simulink model "experiment"  (R2017a)
settings: Solver=ode3  StartTime=0.0  StopTime=inf  FixedStep=Ts_sim  RelTol=1e-3  EnableMultiTasking=on
model workspace (MAT data in the model file):
  SL_ROS_VariableLengthArrays_MaxSizes.CommonInfo.ArrayTruncateAction = 'EmitWarning'
  SL_ROS_VariableLengthArrays_MaxSizes.MsgTypeMap = containers.Map
  SL_ROS_VariableLengthArrays_MaxSizes.MsgTypeMap.serialization.keys = {'std_msgs/Int16MultiArray'}
  SL_ROS_VariableLengthArrays_MaxSizes.MsgTypeMap.serialization.values{1}.PropertyName = 'Data'
  SL_ROS_VariableLengthArrays_MaxSizes.MsgTypeMap.serialization.values{1}.DataType = 'int16'
  SL_ROS_VariableLengthArrays_MaxSizes.MsgTypeMap.serialization.values{1}.MaxLength = 2
  SL_ROS_VariableLengthArrays_MaxSizes.MsgTypeMap.serialization.uniformity = 0
  SL_ROS_VariableLengthArrays_MaxSizes.MsgTypeMap.serialization.keyType = 'char'
  SL_ROS_VariableLengthArrays_MaxSizes.MsgTypeMap.serialization.valueType = 'any'
values from neighbouring files (symbols this model uses):
  b_stop = 2*J*omega_n_stop*xsi_stop    [initializeParameters.m]
  delta_EMG_RT = double(max(EMG_vect_calRT)-min(EMG_vect_calRT))    [initializeParameters.m]
  delta_theta1 = thetaR1_rest - pi/2    (= 0.0728705481978)    [initializeParameters.m]
  EMG2vel_gain = 1*pi    (= 3.14159265359)    [initializeParameters.m]
  emgConst2 = 0    [initializeParameters.m]
  g = 9.81    [initializeParameters.m]
  input_type = 2    [initializeParameters.m]
  k_stop = J*omega_n_stop^2    [initializeParameters.m]
  Ki_vel = 0.75    [initializeParameters.m]
  Kp_vel = 7.5    [initializeParameters.m]
  L_com = tau_lift/(-m_arm*g*cos(thetaR1_lift - delta_theta1))    [initializeParameters.m]
  m1 = (y2_1-y1_1)/(x2_1-x1_1)    (= -1)    [initializeParameters.m]
  m3 = (y2_3-y1_3)/(x2_3-x1_3)    (= -1)    [initializeParameters.m]
  m_arm = 3.45    [initializeParameters.m]
  min_EMG_RT = double(min(EMG_vect_calRT))    [initializeParameters.m]
  q1 = -x1_1*m1 + y1_1    (= 90)    [initializeParameters.m]
  q3 = -x1_3*m3 + y1_3    (= 90)    [initializeParameters.m]
  tau_max_cont = 21    [initializeParameters.m]
  thetaL1_max = 70/180*pi    (= 1.2217304764)    [initializeParameters.m]
  thetaL1_min = -70/180*pi    (= -1.2217304764)    [initializeParameters.m]
  thetaR1_max = 70/180*pi    (= 1.2217304764)    [initializeParameters.m]
  thetaR1_min = -70/180*pi    (= -1.2217304764)    [initializeParameters.m]
undefined symbols (not defined in the file or in its folder): A_butter_cal, A_butter_low, B_butter_cal, B_butter_low, robotics, X, Y, Z
libraries: sm_lib x16, nesl_utility x7, robotlib x3
settings Model: ExtModeTrigDuration=2  Creator=Fred Parietti  LastModifiedBy=jacob
settings DataIOCC: LimitDataPoints=on  SaveFormat=Array
settings OptimizationCC: LifeSpan=1
settings DebuggingCC: UnderspecifiedInitializationDetection=Classic  MergeDetectMultiDrivingBlocksExec=none  SFUnexpectedBacktrackingDiag=warning  SFNoUnconditionalDefaultTransitionDiag=warning  SFExecutionAtInitializationDiag=none
settings HardwareCC: ProdBitPerInt=16  ProdBitPerPointer=8  ProdBitPerSizeT=16  ProdBitPerPtrDiffT=16  ProdLargestAtomicFloat=None  ProdWordSize=8  ProdHWDeviceType=Atmel->AVR
settings ModelReferenceCC: PropagateSignalLabelsOutOfModel=off
settings SFSimCC: MATLABDynamicMemAlloc=off
settings RTWCC: SystemTargetFile=realtime.tlc  GenerateMakefile=off  TemplateMakefile=realtime.tmf  Description=Run on Target Hardware  RTWVerbose=off
settings STFCustomTargetCC: TargetLibSuffix=.a  GenerateSampleERTMain=on  ERTCustomFileBanners=on  SupportNonInlinedSFcns=off  RemoveResetFunc=on  SupportVariableSizeSignals=on  MATLABClassNameForMDSCustomization=Simulink.SoftwareTarget.ERTCustomization  GRTInterface=off  SystemTargetFile=realtime.tlc
settings ERTTargetCC: MultiwordLength=2048  GenerateSampleERTMain=on  ParMdlRefBuildCompliant=off  CompOptLevelCompliant=off  ConcurrentExecutionCompliant=off  CombineOutputUpdateFcns=off  ERTFirstTimeCompliant=off  SupportContinuousTime=on  SupportVariableSizeSignals=on  ModelStepFunctionPrototypeControlCompliant=off  CPPClassGenCompliant=off  UseToolchainInfoCompliant=off  ExtModeTransport=3  ExtModeMexFile=ext_serial_win32_comm_rtt  ExtModeMexArgs=0 1 9600  ERTSrcFileBannerTemplate=realtime_code_template.cgt  ERTHdrFileBannerTemplate=realtime_code_template.cgt  ERTDataSrcFileTemplate=realtime_code_template.cgt  ERTDataHdrFileTemplate=realtime_code_template.cgt  ERTCustomFileTemplate=realtime_file_process.tlc  ConvertIfToSwitch=off  SuppressUnreachableDefaultCases=off
settings ConfigComp: CovMetricSettings=dw  CovHtmlReporting=on  CovSaveCumulativeToWorkspaceVar=on  CovSaveSingleToWorkspaceVar=on  CovExternalEMLEnable=off

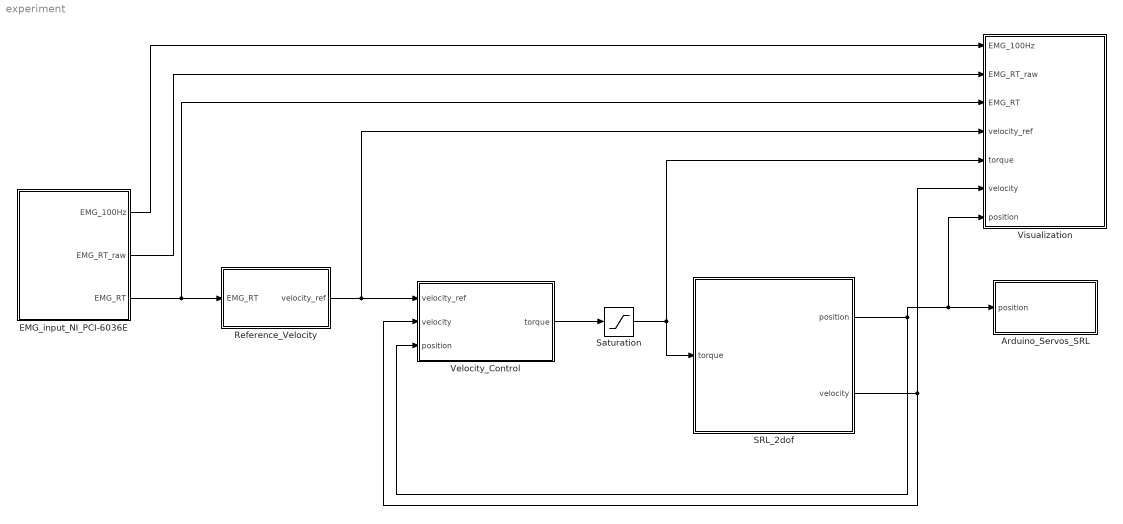
== system experiment ==
  Arduino_Servos_SRL : Subsystem  LoadFcn=robotics.ros.createSimulinkBus(gcs);
  EMG_input_NI_PCI-6036E : Subsystem
  Reference_Velocity : Subsystem
  SRL_2dof : Subsystem
  Saturation : Saturate  UpperLimit=tau_max_cont  LowerLimit=-tau_max_cont
  Velocity_Control : Subsystem
  Visualization : Subsystem
  wires:
  SRL_2dof/1(position) -> Visualization/7(position), Arduino_Servos_SRL/1(position), Velocity_Control/3(position)
  Saturation/1 -> Visualization/5(torque), SRL_2dof/1(torque)
  SRL_2dof/2(velocity) -> Visualization/6(velocity), Velocity_Control/2(velocity)
  Reference_Velocity/1(velocity_ref) -> Velocity_Control/1(velocity_ref), Visualization/4(velocity_ref)
  Velocity_Control/1(torque) -> Saturation/1
  EMG_input_NI_PCI-6036E/3(EMG_RT) -> Visualization/3(EMG_RT), Reference_Velocity/1(EMG_RT)
  EMG_input_NI_PCI-6036E/2(EMG_RT_raw) -> Visualization/2(EMG_RT_raw)
  EMG_input_NI_PCI-6036E/1(EMG_100Hz) -> Visualization/1(EMG_100Hz)

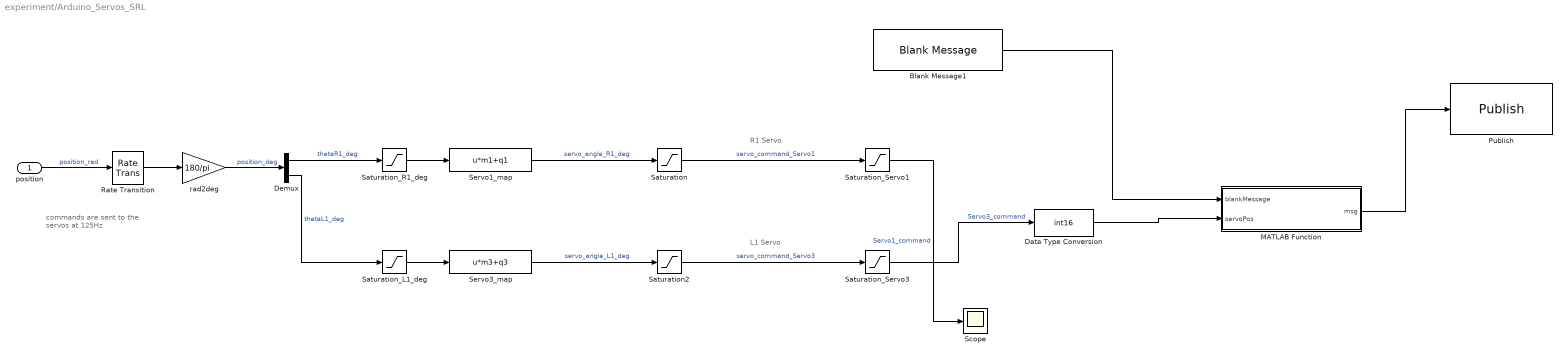
== system experiment/Arduino_Servos_SRL ==
  note: R1 Servo
  note: L1 Servo
  note: commands are sent to the servos at 125Hz
  position : Inport
  Blank Message1 : robotlib/Blank Message  SourceLibraryInfo=This block requires Robotics System Toolbox  messageType=std_msgs/Int16  SampleTime=inf
      settings: SourceProductBaseCode=RO
  Data Type Conversion : DataTypeConversion  OutDataTypeStr=int16  RndMeth=Round
  Demux : Demux  Outputs=2
  MATLAB Function : MATLAB Function  TreatAsAtomicUnit=on
  Publish : robotlib/Publish  SourceLibraryInfo=This block requires Robotics System Toolbox  topicSource=Specify your own  topic=/servoPosEMG  messageType=std_msgs/Int16  messageQueueLength=1
      settings: SourceProductBaseCode=RO
  Rate Transition : RateTransition  Deterministic=off  OutPortSampleTime=0.008
  Saturation : Saturate  UpperLimit=150  LowerLimit=23
  Saturation2 : Saturate  UpperLimit=158  LowerLimit=30
  Saturation_L1_deg : Saturate  UpperLimit=thetaL1_max/pi*180  LowerLimit=thetaL1_min/pi*180
  Saturation_R1_deg : Saturate  UpperLimit=thetaR1_max/pi*180  LowerLimit=thetaR1_min/pi*180
  Saturation_Servo1 : Saturate  UpperLimit=180  LowerLimit=0
  Saturation_Servo3 : Saturate  UpperLimit=180  LowerLimit=0
  Scope : Scope
  Servo1_map : Fcn  Expr=u*m1+q1
  Servo3_map : Fcn  Expr=u*m3+q3
  rad2deg : Gain  Gain=180/pi
  wires:
  position/1 -> Rate Transition/1  "position_rad"
  rad2deg/1 -> Demux/1  "position_deg"
  Demux/1 -> Saturation_R1_deg/1  "thetaR1_deg"
  Servo1_map/1 -> Saturation/1  "servo_angle_R1_deg"
  Demux/2 -> Saturation_L1_deg/1  "thetaL1_deg"
  Servo3_map/1 -> Saturation2/1  "servo_angle_L1_deg"
  Rate Transition/1 -> rad2deg/1
  Saturation/1 -> Saturation_Servo1/1  "servo_command_Servo1"
  Saturation2/1 -> Saturation_Servo3/1  "servo_command_Servo3"
  Saturation_R1_deg/1 -> Servo1_map/1
  Saturation_L1_deg/1 -> Servo3_map/1
  Blank Message1/1 -> MATLAB Function/1(blankMessage)
  Data Type Conversion/1 -> MATLAB Function/2(servoPos)
  MATLAB Function/1(msg) -> Publish/1
  Saturation_Servo3/1 -> Data Type Conversion/1  "Servo3_command"
  Saturation_Servo1/1 -> Scope/1  "Servo1_command"

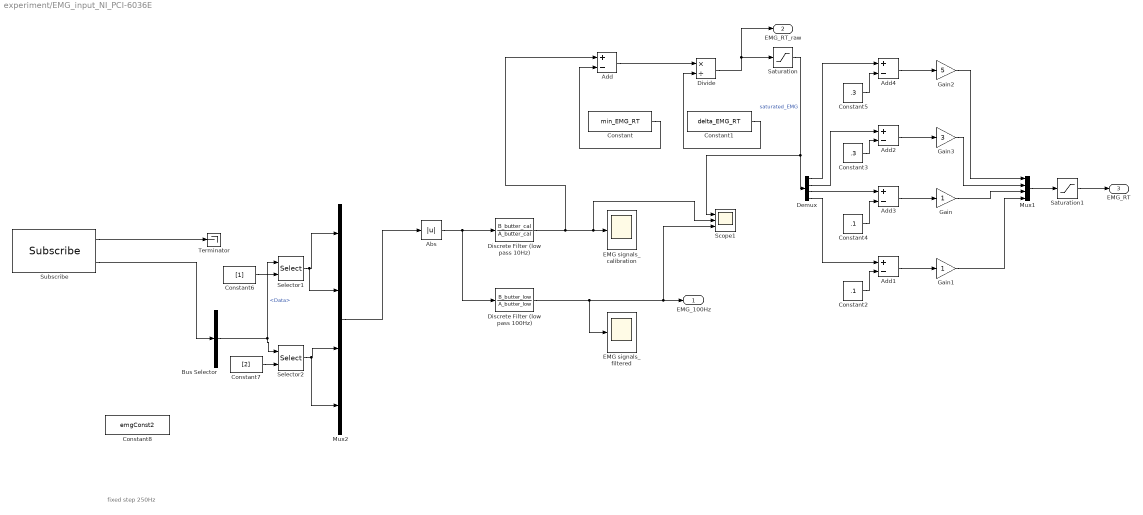
== system experiment/EMG_input_NI_PCI-6036E ==
  note: fixed step 250Hz
  Abs : Abs
  Add{,1..4} (5 alike) : Sum  Inputs=+-
  Bus Selector : BusSelector  OutputSignals=Data
  Constant : Constant  Value=min_EMG_RT
  Constant1 : Constant  Value=delta_EMG_RT
  Constant2 : Constant  Value=.1
  Constant3 : Constant  Value=.3
  Constant4 : Constant  Value=.1
  Constant5 : Constant  Value=.3
  Constant6 : Constant  Value=[1]
  Constant7 : Constant  Value=[2]
  Constant8 : Constant  Value=emgConst2  VectorParams1D=off  OutDataTypeStr=int16
  Demux : Demux
  Discrete Filter (low pass 100Hz) : DiscreteFilter  Numerator=B_butter_low  Denominator=A_butter_low
  Discrete Filter (low pass 10Hz) : DiscreteFilter  Numerator=B_butter_cal  Denominator=A_butter_cal
  Divide : Product  Inputs=*/
  EMG signals_calibration : Scope
  EMG signals_filtered : Scope
  Gain : Gain
  Gain1 : Gain
  Gain2 : Gain  Gain=5
  Gain3 : Gain  Gain=3
  Mux1 : Mux
  Mux2 : Mux
  Saturation : Saturate  UpperLimit=1  LowerLimit=0
  Saturation1 : Saturate  UpperLimit=1  LowerLimit=0
  Scope1 : Scope  NumInputPorts=3
  Selector1 : Selector  IndexOptions=Index vector (port)  Indices=[1 3]  OutputSizes=1
  Selector2 : Selector  IndexOptions=Index vector (port)  Indices=[1 3]  OutputSizes=1
  Subscribe : robotlib/Subscribe  SourceLibraryInfo=This block requires Robotics System Toolbox  topicSource=Select from ROS network  topic=/emgPub  messageType=std_msgs/Int16MultiArray  sampleTime=-1  messageQueueLength=1
      settings: SourceProductBaseCode=RO
  Terminator : Terminator
  EMG_100Hz : Outport
  EMG_RT_raw : Outport  Port=2
  EMG_RT : Outport  Port=3
  wires:
  Constant/1 -> Add/2
  Add/1 -> Divide/1
  Constant1/1 -> Divide/2
  Saturation/1 -> Scope1/1, Demux/1  "saturated_EMG"
  Demux/4 -> Add1/1
  Constant2/1 -> Add1/2
  Demux/1 -> Add4/1
  Add1/1 -> Gain1/1
  Mux1/1 -> Saturation1/1
  Demux/2 -> Add2/1
  Constant3/1 -> Add2/2
  Add2/1 -> Gain3/1
  Saturation1/1 -> EMG_RT/1
  Demux/3 -> Add3/1
  Add3/1 -> Gain/1
  Constant4/1 -> Add3/2
  Constant5/1 -> Add4/2
  Add4/1 -> Gain2/1
  Gain/1 -> Mux1/3
  Gain1/1 -> Mux1/4
  Gain2/1 -> Mux1/1
  Gain3/1 -> Mux1/2
  Discrete Filter (low pass 10Hz)/1 -> Add/1, Scope1/2, EMG signals_calibration/1
  Mux2/1 -> Abs/1
  Abs/1 -> Discrete Filter (low pass 10Hz)/1, Discrete Filter (low pass 100Hz)/1
  Divide/1 -> EMG_RT_raw/1, Saturation/1
  Discrete Filter (low pass 100Hz)/1 -> Scope1/3, EMG_100Hz/1, EMG signals_filtered/1
  Selector2/1 -> Mux2/4, Mux2/3
  Bus Selector/1 -> Selector2/1, Selector1/1  "<Data>"
  Subscribe/2 -> Bus Selector/1
  Constant6/1 -> Selector1/2
  Constant7/1 -> Selector2/2
  Subscribe/1 -> Terminator/1
  Selector1/1 -> Mux2/2, Mux2/1

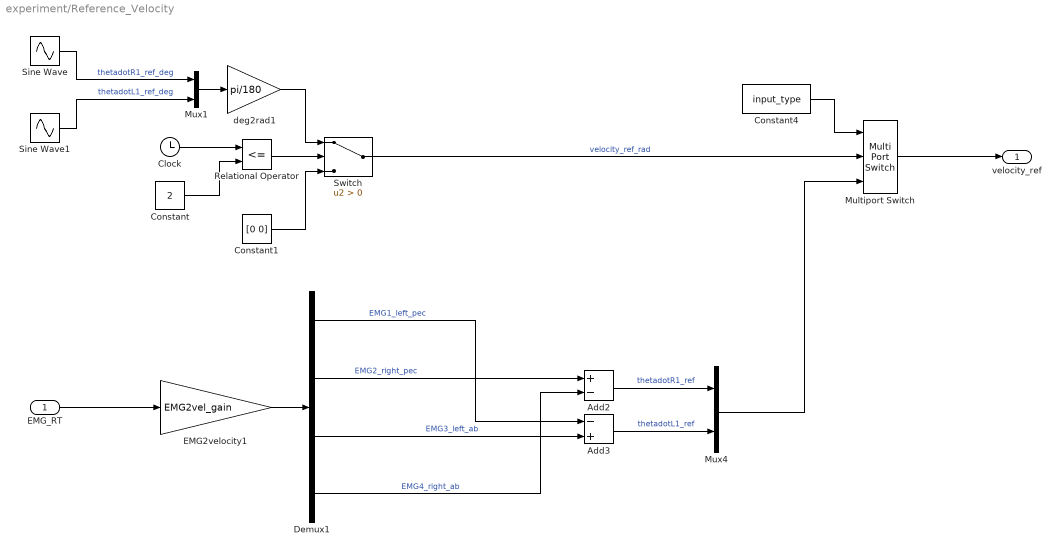
== system experiment/Reference_Velocity ==
  EMG_RT : Inport
  Add2 : Sum  Inputs=+-
  Add3 : Sum  Inputs=-+
  Clock : Clock
  Constant : Constant  Value=2
  Constant1 : Constant  Value=[0 0]
  Constant4 : Constant  Value=input_type
  Demux1 : Demux
  EMG2velocity1 : Gain  Gain=EMG2vel_gain
  Multiport Switch : MultiPortSwitch  Inputs=2
  Mux1 : Mux  Inputs=2
  Mux4 : Mux  Inputs=2
  Relational Operator : RelationalOperator  Operator=<=  OutDataTypeStr=boolean  RndMeth=Nearest
  Sine Wave : Sin  Amplitude=-40  Frequency=2*pi/(4)  SampleTime=0
  Sine Wave1 : Sin  Amplitude=-40  Frequency=2*pi/(4)  SampleTime=0
  Switch : Switch  Criteria=u2 > Threshold
  deg2rad1 : Gain  Gain=pi/180
  velocity_ref : Outport
  wires:
  Sine Wave/1 -> Mux1/1  "thetadotR1_ref_deg"
  Mux1/1 -> deg2rad1/1
  Switch/1 -> Multiport Switch/2  "velocity_ref_rad"
  Clock/1 -> Relational Operator/1
  Constant1/1 -> Switch/3
  Constant/1 -> Relational Operator/2
  Relational Operator/1 -> Switch/2
  deg2rad1/1 -> Switch/1
  Sine Wave1/1 -> Mux1/2  "thetadotL1_ref_deg"
  Constant4/1 -> Multiport Switch/1
  Multiport Switch/1 -> velocity_ref/1
  EMG2velocity1/1 -> Demux1/1
  Demux1/1 -> Add3/1  "EMG1_left_pec"
  Demux1/2 -> Add2/1  "EMG2_right_pec"
  Demux1/3 -> Add3/2  "EMG3_left_ab"
  Demux1/4 -> Add2/2  "EMG4_right_ab"
  Add2/1 -> Mux4/1  "thetadotR1_ref"
  Add3/1 -> Mux4/2  "thetadotL1_ref"
  EMG_RT/1 -> EMG2velocity1/1
  Mux4/1 -> Multiport Switch/3

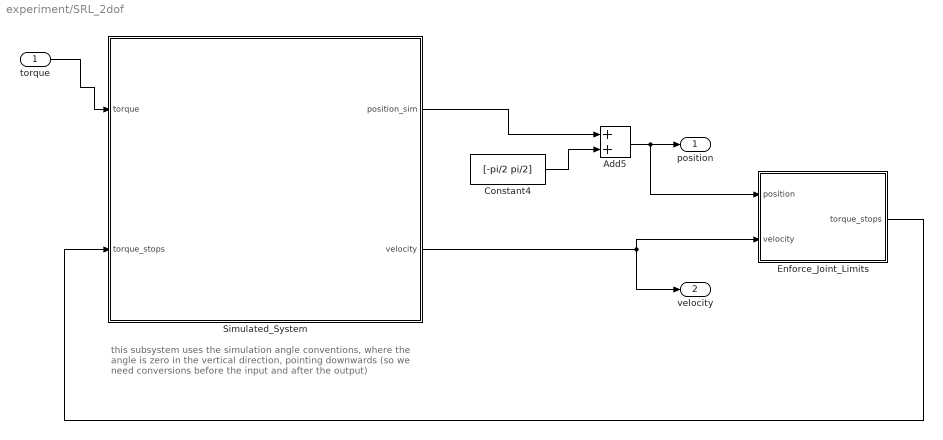
== system experiment/SRL_2dof ==
  note: this subsystem uses the simulation angle conventions, where the
      | angle is zero in the vertical direction, pointing downwards
      | (so we need conversions before the input and after the output)
  torque : Inport
  Add5 : Sum
  Constant4 : Constant  Value=[-pi/2 pi/2]
  Enforce_Joint_Limits : Subsystem
  Simulated_System : Subsystem
  position : Outport
  velocity : Outport  Port=2
  wires:
  Constant4/1 -> Add5/2
  Simulated_System/2(velocity) -> Enforce_Joint_Limits/2(velocity), velocity/1
  torque/1 -> Simulated_System/1(torque)
  Enforce_Joint_Limits/1(torque_stops) -> Simulated_System/2(torque_stops)
  Simulated_System/1(position_sim) -> Add5/1
  Add5/1 -> Enforce_Joint_Limits/1(position), position/1

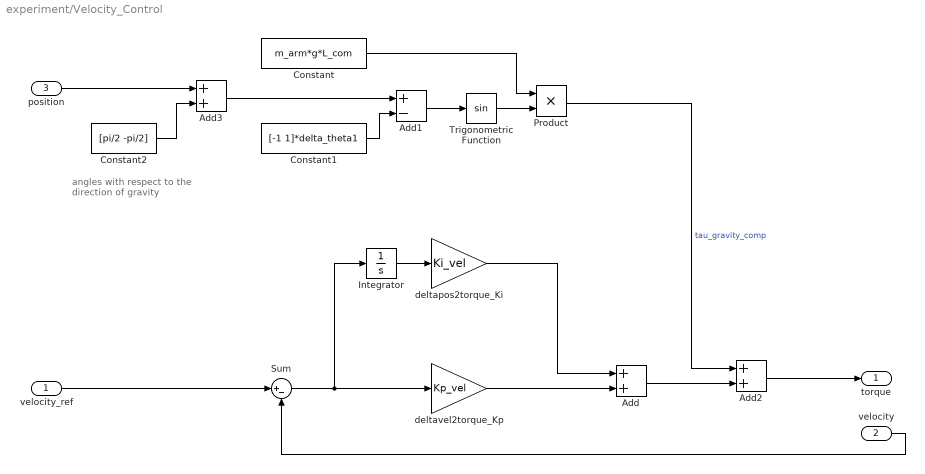
== system experiment/Velocity_Control ==
  note: angles with respect to
      | the direction of gravity
  velocity_ref : Inport
  velocity : Inport  Port=2
  position : Inport  Port=3
  Add : Sum
  Add1 : Sum  Inputs=+-
  Add2 : Sum
  Add3 : Sum
  Constant : Constant  Value=m_arm*g*L_com
  Constant1 : Constant  Value=[-1 1]*delta_theta1
  Constant2 : Constant  Value=[pi/2 -pi/2]
  Integrator : Integrator
  Product : Product
  Sum : Sum  Inputs=|+-
  Trigonometric Function : Trigonometry
  deltapos2torque_Ki : Gain  Gain=Ki_vel
  deltavel2torque_Kp : Gain  Gain=Kp_vel
  torque : Outport
  wires:
  velocity_ref/1 -> Sum/1
  velocity/1 -> Sum/2
  Sum/1 -> deltavel2torque_Kp/1, Integrator/1
  deltavel2torque_Kp/1 -> Add/2
  deltapos2torque_Ki/1 -> Add/1
  Add/1 -> Add2/2
  Integrator/1 -> deltapos2torque_Ki/1
  position/1 -> Add3/1
  Constant1/1 -> Add1/2
  Add1/1 -> Trigonometric Function/1
  Constant/1 -> Product/1
  Trigonometric Function/1 -> Product/2
  Product/1 -> Add2/1  "tau_gravity_comp"
  Add2/1 -> torque/1
  Add3/1 -> Add1/1
  Constant2/1 -> Add3/2

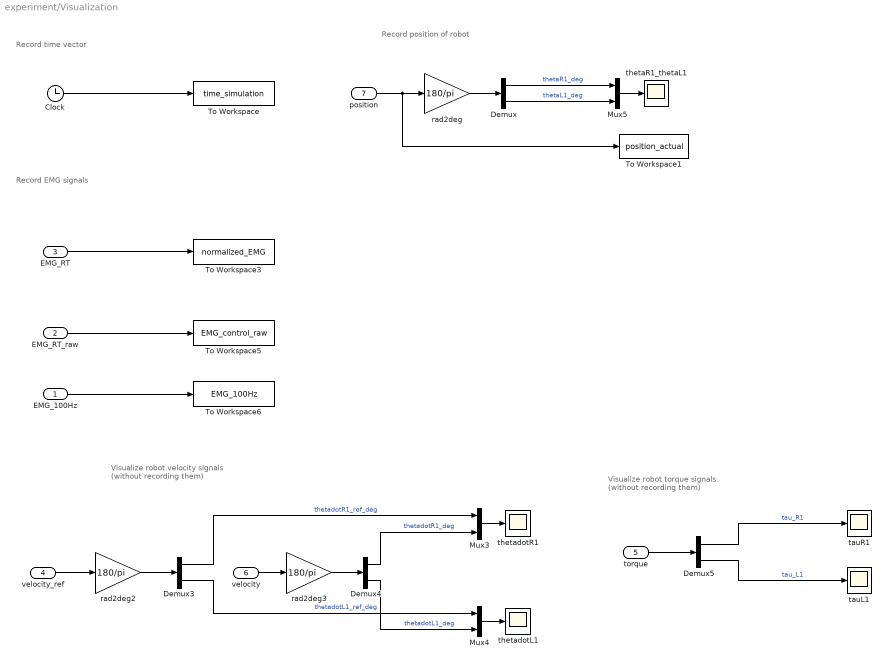
== system experiment/Visualization ==
  note: Record position of robot
  note: Record time vector
  note: Record EMG signals
  note: Visualize robot velocity signals (without recording them)
  note: Visualize robot torque signals (without recording them)
  EMG_100Hz : Inport
  EMG_RT_raw : Inport  Port=2
  EMG_RT : Inport  Port=3
  velocity_ref : Inport  Port=4
  torque : Inport  Port=5
  velocity : Inport  Port=6
  position : Inport  Port=7
  Clock : Clock
  Demux{,3..5} (4 alike) : Demux  Outputs=2
  Mux3 : Mux  Inputs=2
  Mux4 : Mux  Inputs=2
  Mux5 : Mux  Inputs=2
  To Workspace : ToWorkspace  VariableName=time_simulation  SampleTime=-1
  To Workspace1 : ToWorkspace  VariableName=position_actual  SampleTime=-1
  To Workspace3 : ToWorkspace  VariableName=normalized_EMG  SampleTime=-1
  To Workspace5 : ToWorkspace  VariableName=EMG_control_raw  SampleTime=-1
  To Workspace6 : ToWorkspace  VariableName=EMG_100Hz  SampleTime=-1
  rad2deg : Gain  Gain=180/pi
  rad2deg2 : Gain  Gain=180/pi
  rad2deg3 : Gain  Gain=180/pi
  tauL1 : Scope
  tauR1 : Scope
  thetaR1_thetaL1 : Scope
  thetadotL1 : Scope
  thetadotR1 : Scope
  wires:
  torque/1 -> Demux5/1
  Demux5/2 -> tauL1/1  "tau_L1"
  Demux5/1 -> tauR1/1  "tau_R1"
  velocity_ref/1 -> rad2deg2/1
  rad2deg2/1 -> Demux3/1
  velocity/1 -> rad2deg3/1
  Mux3/1 -> thetadotR1/1
  Demux3/1 -> Mux3/1  "thetadotR1_ref_deg"
  rad2deg3/1 -> Demux4/1
  Demux4/1 -> Mux3/2  "thetadotR1_deg"
  Mux4/1 -> thetadotL1/1
  Demux4/2 -> Mux4/2  "thetadotL1_deg"
  Demux3/2 -> Mux4/1  "thetadotL1_ref_deg"
  Clock/1 -> To Workspace/1
  EMG_RT/1 -> To Workspace3/1
  EMG_RT_raw/1 -> To Workspace5/1
  EMG_100Hz/1 -> To Workspace6/1
  position/1 -> rad2deg/1, To Workspace1/1
  rad2deg/1 -> Demux/1
  Demux/2 -> Mux5/2  "thetaL1_deg"
  Demux/1 -> Mux5/1  "thetaR1_deg"
  Mux5/1 -> thetaR1_thetaL1/1

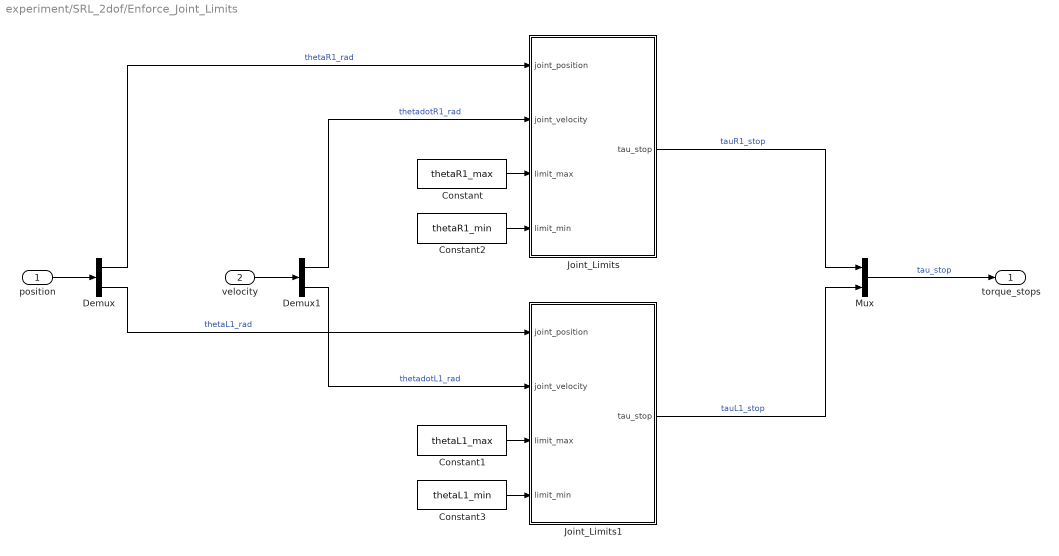
== system experiment/SRL_2dof/Enforce_Joint_Limits ==
  position : Inport
  velocity : Inport  Port=2
  Constant : Constant  Value=thetaR1_max
  Constant1 : Constant  Value=thetaL1_max
  Constant2 : Constant  Value=thetaR1_min
  Constant3 : Constant  Value=thetaL1_min
  Demux : Demux  Outputs=2
  Demux1 : Demux  Outputs=2
  Joint_Limits : Subsystem
  Joint_Limits1 : Subsystem
  Mux : Mux  Inputs=2
  torque_stops : Outport
  wires:
  position/1 -> Demux/1
  velocity/1 -> Demux1/1
  Demux1/1 -> Joint_Limits/2(joint_velocity)  "thetadotR1_rad"
  Constant/1 -> Joint_Limits/3(limit_max)
  Demux/1 -> Joint_Limits/1(joint_position)  "thetaR1_rad"
  Constant2/1 -> Joint_Limits/4(limit_min)
  Joint_Limits/1(tau_stop) -> Mux/1  "tauR1_stop"
  Mux/1 -> torque_stops/1  "tau_stop"
  Demux1/2 -> Joint_Limits1/2(joint_velocity)  "thetadotL1_rad"
  Demux/2 -> Joint_Limits1/1(joint_position)  "thetaL1_rad"
  Constant1/1 -> Joint_Limits1/3(limit_max)
  Constant3/1 -> Joint_Limits1/4(limit_min)
  Joint_Limits1/1(tau_stop) -> Mux/2  "tauL1_stop"

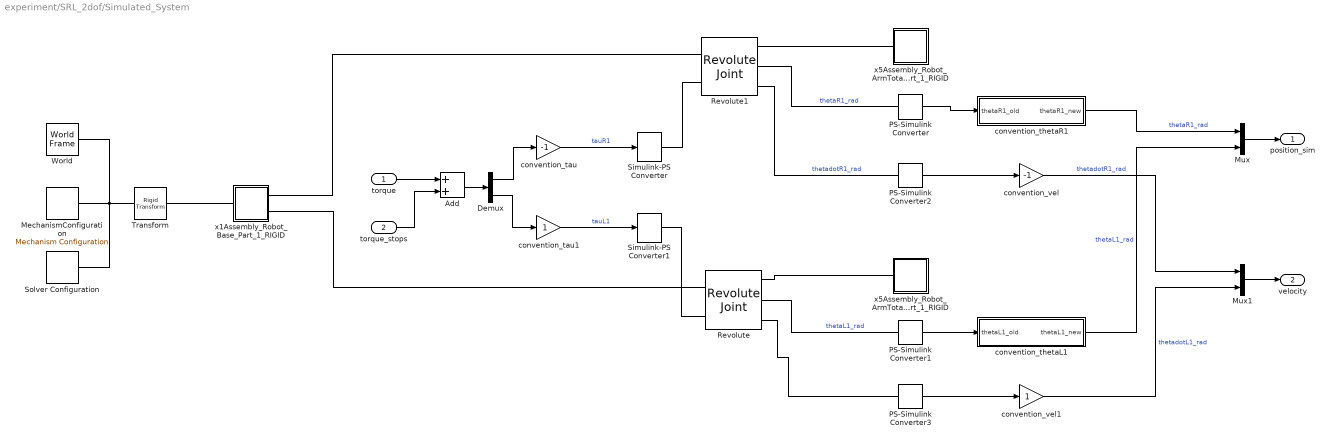
== system experiment/SRL_2dof/Simulated_System ==
  torque : Inport
  torque_stops : Inport  Port=2
  Add : Sum
  Demux : Demux  Outputs=2
  MechanismConfiguration : sm_lib/Utilities/Mechanism Configuration  UniformGravity=Constant  GravityVector=[0 -9.81 0]  GravityUnits=m/s^2  LinearizationDelta=0.001
  Mux : Mux  Inputs=2
  Mux1 : Mux  Inputs=2
  PS-Simulink Converter{,1..3} (4 alike) : nesl_utility/PS-Simulink Converter  PhysicalDomain=network_engine_domain  SubClassName=ps_output  LeftPortType=input  RightPortType=output  PseudoPeriodic=off  Frequencies=[]  Unit=1  AffineConversion=off
  Revolute : sm_lib/Joints/Revolute Joint  SenseConstraintForce=off  SenseConstraintForceX=off  SenseConstraintForceY=off  SenseConstraintForceZ=off  SenseConstraintTorque=off  SenseConstraintTorqueX=off  SenseConstraintTorqueY=off  SenseConstraintTorqueZ=off  SenseTotalForce=off  SenseTotalForceX=off  SenseTotalForceY=off  SenseTotalForceZ=off  SenseTotalTorque=off  SenseTotalTorqueX=off  SenseTotalTorqueY=off  SenseTotalTorqueZ=off  CompositeWrenchDir=FollowerOnBase  CompositeWrenchFrame=BaseFrame  EquilibriumPosition=0  EquilibriumPositionUnits=rad  SpringStiffness=0  SpringStiffnessUnits=m*N/rad  DampingCoefficient=0  DampingCoefficientUnits=m*s*N/rad  TorqueActuationMode=InputTorque  MotionActuationMode=ComputedMotion  SensePosition=on  SenseVelocity=on  SenseAcceleration=off  SenseTorqueForce=off  PositionTargetSpecify=on  PositionTargetPriority=Low  PositionTargetValue=0  PositionTargetValueUnits=deg  VelocityTargetSpecify=off  VelocityTargetPriority=High  VelocityTargetValue=0  VelocityTargetValueUnits=deg/s
  Revolute1 : sm_lib/Joints/Revolute Joint  SenseConstraintForce=off  SenseConstraintForceX=off  SenseConstraintForceY=off  SenseConstraintForceZ=off  SenseConstraintTorque=off  SenseConstraintTorqueX=off  SenseConstraintTorqueY=off  SenseConstraintTorqueZ=off  SenseTotalForce=off  SenseTotalForceX=off  SenseTotalForceY=off  SenseTotalForceZ=off  SenseTotalTorque=off  SenseTotalTorqueX=off  SenseTotalTorqueY=off  SenseTotalTorqueZ=off  CompositeWrenchDir=FollowerOnBase  CompositeWrenchFrame=BaseFrame  EquilibriumPosition=0  EquilibriumPositionUnits=rad  SpringStiffness=0  SpringStiffnessUnits=m*N/rad  DampingCoefficient=0  DampingCoefficientUnits=m*s*N/rad  TorqueActuationMode=InputTorque  MotionActuationMode=ComputedMotion  SensePosition=on  SenseVelocity=on  SenseAcceleration=off  SenseTorqueForce=off  PositionTargetSpecify=on  PositionTargetPriority=Low  PositionTargetValue=0  PositionTargetValueUnits=deg  VelocityTargetSpecify=off  VelocityTargetPriority=High  VelocityTargetValue=0  VelocityTargetValueUnits=deg/s
  Simulink-PS Converter : nesl_utility/Simulink-PS Converter  PhysicalDomain=network_engine_domain  SubClassName=ps_input  LeftPortType=input  RightPortType=output  PseudoPeriodic=off  Frequencies=[]  NoiseDistribution=none  NoiseParameters=[]  Unit=1  AffineConversion=off  FilteringAndDerivatives=zero  SimscapeFilterOrder=1  InputFilterTimeConstant=0.001  UdotUserProvided=1
  Simulink-PS Converter1 : nesl_utility/Simulink-PS Converter  PhysicalDomain=network_engine_domain  SubClassName=ps_input  LeftPortType=input  RightPortType=output  PseudoPeriodic=off  Frequencies=[]  NoiseDistribution=none  NoiseParameters=[]  Unit=1  AffineConversion=off  FilteringAndDerivatives=zero  SimscapeFilterOrder=1  InputFilterTimeConstant=0.001  UdotUserProvided=1
  Solver Configuration : nesl_utility/Solver Configuration  PhysicalDomain=network_engine_domain  SubClassName=solver  LeftPortType=input  RightPortType=generic  Accelerate=off  Tones=[]  Harmonics=[]  SimulateNoise=off  Profile=off  UseLocalSampling=off  EnableSwitchedLinearOptims=on  FrequencyDomain=off  UseCCode=off  RelTol=0.001  AbsTol=1e-06  MinStep=1e-09  ToWorkspace=off  RevertToSquareIcSolve=off  NumHomotopyIterations=100  PhasorMode=off  PhasorModeNumHarmonics=1  OverrideAbsTol=off  DoDC=off  ResidualTolerance=1e-09  UseLocalSolver=off  LocalSolverChoice=NE_BACKWARD_EULER_ADVANCER  LocalSolverSampleTime=0.001  DoFixedCost=off  MaxNonlinIter=3  MaxModeIter=2  LinearAlgebra=Sparse  DelaysMemoryBudget=1024  AutomaticFiltering=on  FilteringTimeConstant=0.001
  Transform : sm_lib/Frames and Transforms/Rigid Transform  TranslationMethod=Cartesian  TranslationStandardOffset=0  TranslationLengthUnit=mm  TranslationStandardAxis=+Z  TranslationCartesianOffset=[-131.68773658972694 0 0]  TranslationROffset=0  TranslationROffsetUnits=m  TranslationZOffset=0  TranslationZOffsetUnits=m  TranslationThetaOffset=0  TranslationThetaOffsetUnits=deg  RotationMethod=ArbitraryAxis  RotationAngleUnits=rad  RotationStandardAxis=+Z  RotationAngle=0  RotationArbitraryAxis=[0 0 0]  FollAlignAxisA=+X  BaseAlignAxisA=+Y  FollAlignAxisB=+Y  BaseAlignAxisB=+Z  RotationSequenceAxes=FollowerAxes  RotationSequence=XYX  RotationSequenceAngles=[0 0 0]  RotationSequenceAnglesUnits=deg  RotationMatrix=[1 0 0; 0 1 0; 0 0 1]
  World : sm_lib/Frames and Transforms/World Frame
  convention_tau : Gain  Gain=-1
  convention_tau1 : Gain
  convention_thetaL1 : Subsystem
  convention_thetaR1 : Subsystem
  convention_vel : Gain  Gain=-1
  convention_vel1 : Gain
  x1Assembly_Robot_Base_Part_1_RIGID : Subsystem
  x5Assembly_Robot_ArmTotalShoulder_L_Part_1_RIGID : Subsystem
  x5Assembly_Robot_ArmTotalShoulder_R_Part_1_RIGID : Subsystem
  position_sim : Outport
  velocity : Outport  Port=2
  wires:
  PS-Simulink Converter/1 -> convention_thetaR1/1(thetaR1_old)
  PS-Simulink Converter1/1 -> convention_thetaL1/1(thetaL1_old)
  Mux/1 -> position_sim/1
  torque/1 -> Add/1
  Demux/1 -> convention_tau/1
  Demux/2 -> convention_tau1/1
  Mux1/1 -> velocity/1
  PS-Simulink Converter2/1 -> convention_vel/1
  PS-Simulink Converter3/1 -> convention_vel1/1
  Add/1 -> Demux/1
  torque_stops/1 -> Add/2
  convention_thetaR1/1(thetaR1_new) -> Mux/1  "thetaR1_rad"
  convention_thetaL1/1(thetaL1_new) -> Mux/2  "thetaL1_rad"
  convention_vel/1 -> Mux1/1  "thetadotR1_rad"
  convention_vel1/1 -> Mux1/2  "thetadotL1_rad"
  convention_tau/1 -> Simulink-PS Converter/1  "tauR1"
  convention_tau1/1 -> Simulink-PS Converter1/1  "tauL1"
  connections:
  PS-Simulink Converter/LConn1 -- Revolute1/RConn2  "thetaR1_rad"
  Revolute/RConn2 -- PS-Simulink Converter1/LConn1  "thetaL1_rad"
  Revolute/LConn1 -- x1Assembly_Robot_Base_Part_1_RIGID/RConn2
  Revolute/RConn1 -- x5Assembly_Robot_ArmTotalShoulder_L_Part_1_RIGID/LConn1
  Transform/RConn1 -- x1Assembly_Robot_Base_Part_1_RIGID/LConn1
  Revolute1/LConn1 -- x1Assembly_Robot_Base_Part_1_RIGID/RConn1
  Revolute1/RConn1 -- x5Assembly_Robot_ArmTotalShoulder_R_Part_1_RIGID/LConn1
  Simulink-PS Converter/RConn1 -- Revolute1/LConn2
  Revolute/LConn2 -- Simulink-PS Converter1/RConn1
  Revolute1/RConn3 -- PS-Simulink Converter2/LConn1  "thetadotR1_rad"
  MechanismConfiguration/RConn1 -- Transform/LConn1 -- Solver Configuration/RConn1 -- World/RConn1
  Revolute/RConn3 -- PS-Simulink Converter3/LConn1

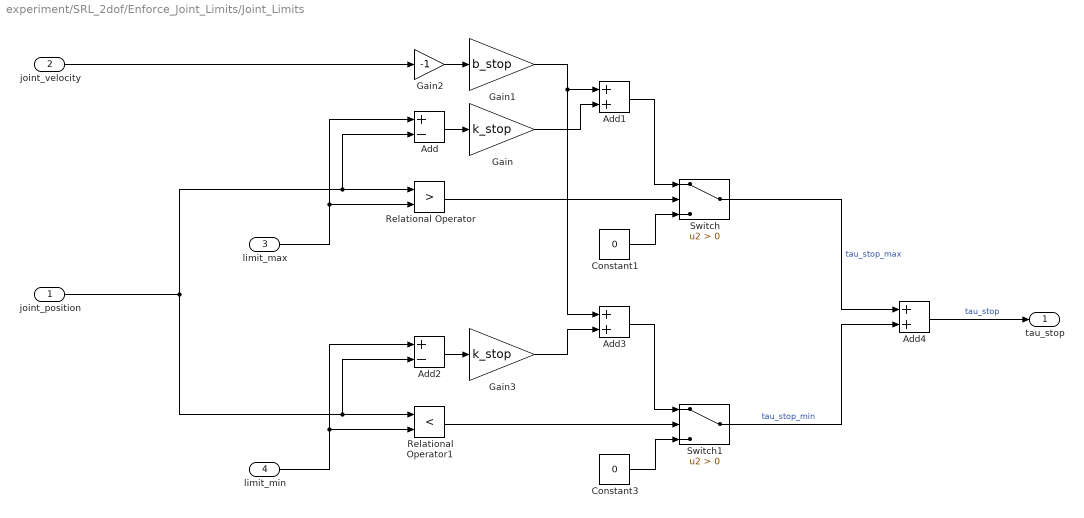
== system experiment/SRL_2dof/Enforce_Joint_Limits/Joint_Limits ==
  joint_position : Inport
  joint_velocity : Inport  Port=2
  limit_max : Inport  Port=3
  limit_min : Inport  Port=4
  Add : Sum  Inputs=+-
  Add1 : Sum
  Add2 : Sum  Inputs=+-
  Add3 : Sum
  Add4 : Sum
  Constant1 : Constant  Value=0
  Constant3 : Constant  Value=0
  Gain : Gain  Gain=k_stop
  Gain1 : Gain  Gain=b_stop
  Gain2 : Gain  Gain=-1
  Gain3 : Gain  Gain=k_stop
  Relational Operator : RelationalOperator  Operator=>  OutDataTypeStr=boolean  RndMeth=Nearest
  Relational Operator1 : RelationalOperator  Operator=<  OutDataTypeStr=boolean  RndMeth=Nearest
  Switch : Switch  Criteria=u2 > Threshold
  Switch1 : Switch  Criteria=u2 > Threshold
  tau_stop : Outport
  wires:
  Gain2/1 -> Gain1/1
  joint_velocity/1 -> Gain2/1
  Gain1/1 -> Add3/1, Add1/1
  limit_max/1 -> Relational Operator/2, Add/1
  Relational Operator/1 -> Switch/2
  Constant1/1 -> Switch/3
  Gain/1 -> Add1/2
  Add/1 -> Gain/1
  limit_min/1 -> Relational Operator1/2, Add2/1
  Constant3/1 -> Switch1/3
  Add1/1 -> Switch/1
  Add4/1 -> tau_stop/1  "tau_stop"
  Relational Operator1/1 -> Switch1/2
  Add2/1 -> Gain3/1
  joint_position/1 -> Add2/2, Relational Operator1/1, Add/2, Relational Operator/1
  Gain3/1 -> Add3/2
  Add3/1 -> Switch1/1
  Switch/1 -> Add4/1  "tau_stop_max"
  Switch1/1 -> Add4/2  "tau_stop_min"

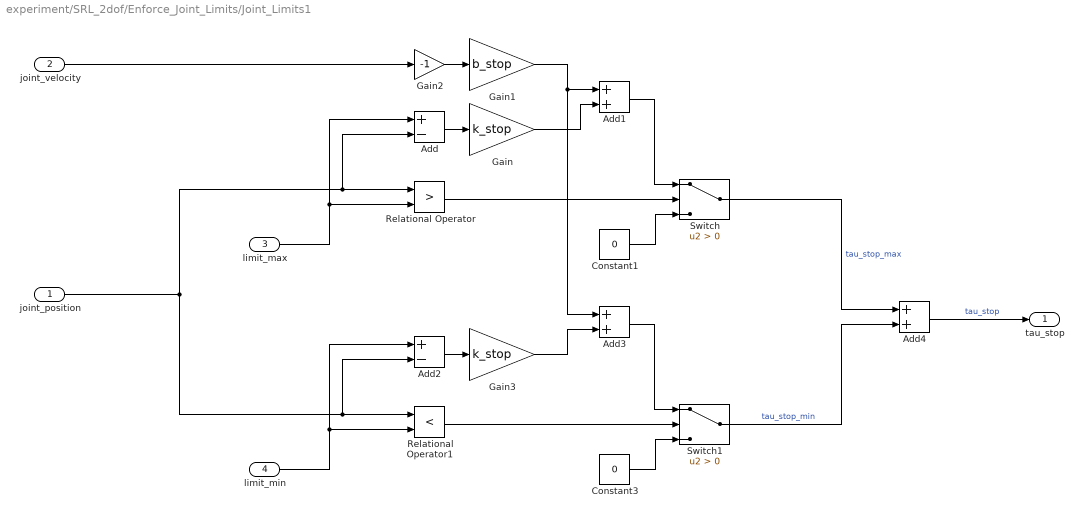
== system experiment/SRL_2dof/Enforce_Joint_Limits/Joint_Limits1 ==
  joint_position : Inport
  joint_velocity : Inport  Port=2
  limit_max : Inport  Port=3
  limit_min : Inport  Port=4
  Add : Sum  Inputs=+-
  Add1 : Sum
  Add2 : Sum  Inputs=+-
  Add3 : Sum
  Add4 : Sum
  Constant1 : Constant  Value=0
  Constant3 : Constant  Value=0
  Gain : Gain  Gain=k_stop
  Gain1 : Gain  Gain=b_stop
  Gain2 : Gain  Gain=-1
  Gain3 : Gain  Gain=k_stop
  Relational Operator : RelationalOperator  Operator=>  OutDataTypeStr=boolean  RndMeth=Nearest
  Relational Operator1 : RelationalOperator  Operator=<  OutDataTypeStr=boolean  RndMeth=Nearest
  Switch : Switch  Criteria=u2 > Threshold
  Switch1 : Switch  Criteria=u2 > Threshold
  tau_stop : Outport
  wires:
  Gain2/1 -> Gain1/1
  joint_velocity/1 -> Gain2/1
  Gain1/1 -> Add3/1, Add1/1
  limit_max/1 -> Relational Operator/2, Add/1
  Relational Operator/1 -> Switch/2
  Constant1/1 -> Switch/3
  Gain/1 -> Add1/2
  Add/1 -> Gain/1
  limit_min/1 -> Relational Operator1/2, Add2/1
  Constant3/1 -> Switch1/3
  Add1/1 -> Switch/1
  Add4/1 -> tau_stop/1  "tau_stop"
  Relational Operator1/1 -> Switch1/2
  Add2/1 -> Gain3/1
  joint_position/1 -> Add2/2, Relational Operator1/1, Add/2, Relational Operator/1
  Gain3/1 -> Add3/2
  Add3/1 -> Switch1/1
  Switch/1 -> Add4/1  "tau_stop_max"
  Switch1/1 -> Add4/2  "tau_stop_min"

== system experiment/SRL_2dof/Simulated_System/convention_thetaL1 ==
  thetaL1_old : Inport
  Add : Sum  Inputs=+-
  Constant : Constant  Value=pi/2
  thetaL1_new : Outport
  wires:
  thetaL1_old/1 -> Add/1
  Constant/1 -> Add/2
  Add/1 -> thetaL1_new/1

== system experiment/SRL_2dof/Simulated_System/convention_thetaR1 ==
  thetaR1_old : Inport
  Add : Sum  Inputs=+-
  Constant : Constant  Value=pi/2
  thetaR1_new : Outport
  wires:
  Add/1 -> thetaR1_new/1
  Constant/1 -> Add/1
  thetaR1_old/1 -> Add/2

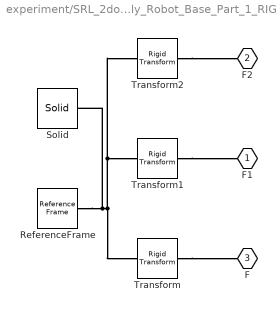
== system experiment/SRL_2dof/Simulated_System/x1Assembly_Robot_Base_Part_1_RIGID ==
  ReferenceFrame : sm_lib/Frames and Transforms/Reference Frame
  Solid : sm_lib/Body Elements/Solid  InertiaType=Custom  Mass=4.0668031749253819*1.07  MassUnits=kg  CenterOfMass=[132.10631157101429 232.16373002543398 333.07087877338296]  CenterOfMassUnits=mm  MomentsOfInertia=[10635.813337617805 181856.04319404627 175955.74045389923]*1.07  MomentsOfInertiaUnits=kg*mm^2  ProductsOfInertia=[1070.5712168307796 -231.15524464943257 317.20376256591442]*1.07  ProductsOfInertiaUnits=kg*mm^2  DensityBased=on  Density=1000  DensityUnits=kg/(m^3)  DoExposeReferenceFrame=on  SerializedFrames=<Frames/>  GraphicType=FromGeometry  MarkerShape=Sphere  MarkerSize=10  MarkerSizeUnits=m  GraphicVisPropType=SimpleVisualProperties  GraphicDiffuseColor=[0.6 0.8 1.0]  GraphicSpecularColor=[0.5 0.5 0.5 1.0]  GraphicAmbientColor=[0.15 0.15 0.15 1.0]  GraphicEmissiveColor=[0.0 0.0 0.0 1.0]  GraphicShininess=75  GraphicOpacity=1  GeometryShape=FromFile  RectangleSize=[1 1]  RectangleSizeUnits=m  BrickDimensions=[1 1 1]  BrickDimensionUnits=m  CylinderRadius=1  CylinderRadiusUnits=m  CylinderLength=1  CylinderLengthUnits=m  SphereRadius=1  SphereRadiusUnits=m  EllipsoidRadii=[1 1 1]  EllipsoidRadiiUnits=m  ExtrusionCrossSection=[1 1; -1 1; -1 -1; 1 -1]  ExtrusionCrossSectionUnits=m  ExtrusionLength=1  ExtrusionLengthUnits=m  PolygonNumSides=3  PolygonOuterRadius=1  PolygonOuterRadiusUnits=m  ExtGeomFileType=STL  ExtGeomFileName=1Assembly_Robot_Base_Part_Default_sldprt.STL  ExtGeomFileUnits=mm  RevolutionCrossSection=[1 1; 1 -1; 2 -1; 2 1]  RevolutionCrossSectionUnits=m  RevolutionExtent=Full  RevolutionAngle=180  RevolutionAngleUnits=deg
  Transform : sm_lib/Frames and Transforms/Rigid Transform  TranslationMethod=Cartesian  TranslationStandardOffset=0  TranslationLengthUnit=mm  TranslationStandardAxis=+Z  TranslationCartesianOffset=[417.19188514110454 220.50618817795819 393.1157122563057]  TranslationROffset=0  TranslationROffsetUnits=m  TranslationZOffset=0  TranslationZOffsetUnits=m  TranslationThetaOffset=0  TranslationThetaOffsetUnits=deg  RotationMethod=ArbitraryAxis  RotationAngleUnits=rad  RotationStandardAxis=+Z  RotationAngle=2.0943951023931948  RotationArbitraryAxis=[0.57735026918962584 0.57735026918962562 0.57735026918962595]  FollAlignAxisA=+X  BaseAlignAxisA=+Y  FollAlignAxisB=+Y  BaseAlignAxisB=+Z  RotationSequenceAxes=FollowerAxes  RotationSequence=XYX  RotationSequenceAngles=[0 0 0]  RotationSequenceAnglesUnits=deg  RotationMatrix=[1 0 0; 0 1 0; 0 0 1]
  Transform1 : sm_lib/Frames and Transforms/Rigid Transform  TranslationMethod=Cartesian  TranslationStandardOffset=0  TranslationLengthUnit=mm  TranslationStandardAxis=+Z  TranslationCartesianOffset=[0 0 0]  TranslationROffset=0  TranslationROffsetUnits=m  TranslationZOffset=0  TranslationZOffsetUnits=m  TranslationThetaOffset=0  TranslationThetaOffsetUnits=deg  RotationMethod=ArbitraryAxis  RotationAngleUnits=rad  RotationStandardAxis=+Z  RotationAngle=0  RotationArbitraryAxis=[0 0 0]  FollAlignAxisA=+X  BaseAlignAxisA=+Y  FollAlignAxisB=+Y  BaseAlignAxisB=+Z  RotationSequenceAxes=FollowerAxes  RotationSequence=XYX  RotationSequenceAngles=[0 0 0]  RotationSequenceAnglesUnits=deg  RotationMatrix=[1 0 0; 0 1 0; 0 0 1]
  Transform2 : sm_lib/Frames and Transforms/Rigid Transform  TranslationMethod=Cartesian  TranslationStandardOffset=0  TranslationLengthUnit=mm  TranslationStandardAxis=+Z  TranslationCartesianOffset=[-161.81641196165057 220.50618817795822 393.1157122563057]  TranslationROffset=0  TranslationROffsetUnits=m  TranslationZOffset=0  TranslationZOffsetUnits=m  TranslationThetaOffset=0  TranslationThetaOffsetUnits=deg  RotationMethod=ArbitraryAxis  RotationAngleUnits=rad  RotationStandardAxis=+Z  RotationAngle=2.0943951023931957  RotationArbitraryAxis=[0.57735026918962573 0.57735026918962573 0.57735026918962562]  FollAlignAxisA=+X  BaseAlignAxisA=+Y  FollAlignAxisB=+Y  BaseAlignAxisB=+Z  RotationSequenceAxes=FollowerAxes  RotationSequence=XYX  RotationSequenceAngles=[0 0 0]  RotationSequenceAnglesUnits=deg  RotationMatrix=[1 0 0; 0 1 0; 0 0 1]
  F1 : PMIOPort  Port=1  Side=Left
  F2 : PMIOPort  Port=2  Side=Right
  F : PMIOPort  Port=3  Side=Right
  connections:
  Solid/RConn1 -- ReferenceFrame/RConn1 -- Transform1/LConn1 -- Transform2/LConn1 -- Transform/LConn1
  Transform/RConn1 -- F/RConn1
  Transform1/RConn1 -- F1/RConn1
  Transform2/RConn1 -- F2/RConn1

== system experiment/SRL_2dof/Simulated_System/x5Assembly_Robot_ArmTotalShoulder_L_Part_1_RIGID ==
  ReferenceFrame : sm_lib/Frames and Transforms/Reference Frame
  Solid : sm_lib/Body Elements/Solid  InertiaType=Custom  Mass=4.748465440366882*0.73  MassUnits=kg  CenterOfMass=[61.561810743979279 194.10237852765343 -263.38581919268194]  CenterOfMassUnits=mm  MomentsOfInertia=[483895.75033506181 471809.67555491626 13215.927467730489]*0.73  MomentsOfInertiaUnits=kg*mm^2  ProductsOfInertia=[39022.626043403077 -558.59126803807874 128.82174045340341]*0.73  ProductsOfInertiaUnits=kg*mm^2  DensityBased=on  Density=1000  DensityUnits=kg/(m^3)  DoExposeReferenceFrame=on  SerializedFrames=<Frames/>  GraphicType=FromGeometry  MarkerShape=Sphere  MarkerSize=10  MarkerSizeUnits=m  GraphicVisPropType=SimpleVisualProperties  GraphicDiffuseColor=[0.6 1.0 0.6]  GraphicSpecularColor=[0.5 0.5 0.5 1.0]  GraphicAmbientColor=[0.15 0.15 0.15 1.0]  GraphicEmissiveColor=[0.0 0.0 0.0 1.0]  GraphicShininess=75  GraphicOpacity=1  GeometryShape=FromFile  RectangleSize=[1 1]  RectangleSizeUnits=m  BrickDimensions=[1 1 1]  BrickDimensionUnits=m  CylinderRadius=1  CylinderRadiusUnits=m  CylinderLength=1  CylinderLengthUnits=m  SphereRadius=1  SphereRadiusUnits=m  EllipsoidRadii=[1 1 1]  EllipsoidRadiiUnits=m  ExtrusionCrossSection=[1 1; -1 1; -1 -1; 1 -1]  ExtrusionCrossSectionUnits=m  ExtrusionLength=1  ExtrusionLengthUnits=m  PolygonNumSides=3  PolygonOuterRadius=1  PolygonOuterRadiusUnits=m  ExtGeomFileType=STL  ExtGeomFileName=5Assembly_Robot_ArmTotalShoulder_L_Part_Default_sldprt.STL  ExtGeomFileUnits=mm  RevolutionCrossSection=[1 1; 1 -1; 2 -1; 2 1]  RevolutionCrossSectionUnits=m  RevolutionExtent=Full  RevolutionAngle=180  RevolutionAngleUnits=deg
  Transform : sm_lib/Frames and Transforms/Rigid Transform  TranslationMethod=Cartesian  TranslationStandardOffset=0  TranslationLengthUnit=mm  TranslationStandardAxis=+Z  TranslationCartesianOffset=[103.05324778099992 163.04696183251519 162.03237626739079]  TranslationROffset=0  TranslationROffsetUnits=m  TranslationZOffset=0  TranslationZOffsetUnits=m  TranslationThetaOffset=0  TranslationThetaOffsetUnits=deg  RotationMethod=ArbitraryAxis  RotationAngleUnits=rad  RotationStandardAxis=+Z  RotationAngle=2.0943951023931962  RotationArbitraryAxis=[-0.57735026918962595 -0.57735026918962606 0.5773502691896254]  FollAlignAxisA=+X  BaseAlignAxisA=+Y  FollAlignAxisB=+Y  BaseAlignAxisB=+Z  RotationSequenceAxes=FollowerAxes  RotationSequence=XYX  RotationSequenceAngles=[0 0 0]  RotationSequenceAnglesUnits=deg  RotationMatrix=[1 0 0; 0 1 0; 0 0 1]
  F : PMIOPort  Port=1  Side=Left
  connections:
  Solid/RConn1 -- ReferenceFrame/RConn1 -- Transform/LConn1
  Transform/RConn1 -- F/RConn1

== system experiment/SRL_2dof/Simulated_System/x5Assembly_Robot_ArmTotalShoulder_R_Part_1_RIGID ==
  ReferenceFrame : sm_lib/Frames and Transforms/Reference Frame
  Solid : sm_lib/Body Elements/Solid  InertiaType=Custom  Mass=4.748465440366882*0.73  MassUnits=kg  CenterOfMass=[60.770137405721343 194.10237852765343 587.45016030684508]  CenterOfMassUnits=mm  MomentsOfInertia=[483897.4125423212 471814.44083118526 13219.030536739923]*0.73  MomentsOfInertiaUnits=kg*mm^2  ProductsOfInertia=[-39022.554479998478 1108.8919330033223 171.58557556982879]*0.73  ProductsOfInertiaUnits=kg*mm^2  DensityBased=on  Density=1000  DensityUnits=kg/(m^3)  DoExposeReferenceFrame=on  SerializedFrames=<Frames/>  GraphicType=FromGeometry  MarkerShape=Sphere  MarkerSize=10  MarkerSizeUnits=m  GraphicVisPropType=SimpleVisualProperties  GraphicDiffuseColor=[0.6 1.0 0.6]  GraphicSpecularColor=[0.5 0.5 0.5 1.0]  GraphicAmbientColor=[0.15 0.15 0.15 1.0]  GraphicEmissiveColor=[0.0 0.0 0.0 1.0]  GraphicShininess=75  GraphicOpacity=1  GeometryShape=FromFile  RectangleSize=[1 1]  RectangleSizeUnits=m  BrickDimensions=[1 1 1]  BrickDimensionUnits=m  CylinderRadius=1  CylinderRadiusUnits=m  CylinderLength=1  CylinderLengthUnits=m  SphereRadius=1  SphereRadiusUnits=m  EllipsoidRadii=[1 1 1]  EllipsoidRadiiUnits=m  ExtrusionCrossSection=[1 1; -1 1; -1 -1; 1 -1]  ExtrusionCrossSectionUnits=m  ExtrusionLength=1  ExtrusionLengthUnits=m  PolygonNumSides=3  PolygonOuterRadius=1  PolygonOuterRadiusUnits=m  ExtGeomFileType=STL  ExtGeomFileName=5Assembly_Robot_ArmTotalShoulder_R_Part_Default_sldprt.STL  ExtGeomFileUnits=mm  RevolutionCrossSection=[1 1; 1 -1; 2 -1; 2 1]  RevolutionCrossSectionUnits=m  RevolutionExtent=Full  RevolutionAngle=180  RevolutionAngleUnits=deg
  Transform : sm_lib/Frames and Transforms/Rigid Transform  TranslationMethod=Cartesian  TranslationStandardOffset=0  TranslationLengthUnit=mm  TranslationStandardAxis=+Z  TranslationCartesianOffset=[95.053247780999769 163.04696183251394 162.03237626738857]  TranslationROffset=0  TranslationROffsetUnits=m  TranslationZOffset=0  TranslationZOffsetUnits=m  TranslationThetaOffset=0  TranslationThetaOffsetUnits=deg  RotationMethod=ArbitraryAxis  RotationAngleUnits=rad  RotationStandardAxis=+Z  RotationAngle=2.0943951023931948  RotationArbitraryAxis=[0.57735026918962573 0.57735026918962562 0.57735026918962595]  FollAlignAxisA=+X  BaseAlignAxisA=+Y  FollAlignAxisB=+Y  BaseAlignAxisB=+Z  RotationSequenceAxes=FollowerAxes  RotationSequence=XYX  RotationSequenceAngles=[0 0 0]  RotationSequenceAnglesUnits=deg  RotationMatrix=[1 0 0; 0 1 0; 0 0 1]
  F : PMIOPort  Port=1  Side=Left
  connections:
  Solid/RConn1 -- ReferenceFrame/RConn1 -- Transform/LConn1
  Transform/RConn1 -- F/RConn1

== matlab function experiment/Arduino_Servos_SRL/MATLAB Function ==
  data: blankMessage input; msg output Bus: SL_Bus_experiment_std_msgs_Int16; servoPos input
function msg = createMessage(blankMessage,servoPos)

msg = blankMessage;
% msg.Layout.DataOffset = uint32(0);
% msg.Layout.Dim(1).Size = uint32(1);
% msg.Layout.Dim(1).Stride = uint32(1);

msg.Data = servoPos;
